simulink model "DegradationParameterIResistor"  (R2021a)
settings: Solver=VariableStepAuto  StartTime=0.0  StopTime=10.0  RelTol=1e-3
undefined symbols (not defined in the file or in its folder): Ires_resistance_adjustment
libraries: PB_Library_Master_Working x2
settings Model: Creator=sfaulk  LastModifiedBy=sfaulk

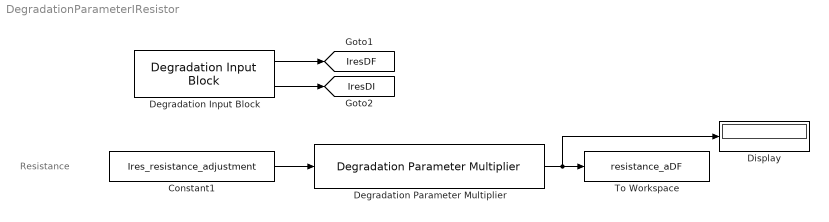
== system DegradationParameterIResistor ==
  note: Resistance
  Constant1 : Constant  Value=Ires_resistance_adjustment
  Degradation Input Block : PB_Library_Master_Working/Degradation Input Block  SystemSampleTime=-1  VariantActivationTime=update diagram  Latency=0  AutoFrameSizeCalculation=off
      link override Degradation Input Value: Value=Ires_degradation_input
  Degradation Parameter Multiplier : PB_Library_Master_Working/Degradation Parameter Multiplier  SystemSampleTime=-1  VariantActivationTime=update diagram  Latency=0  AutoFrameSizeCalculation=off
      link override From14: GotoTag=IresDF
      link override From15: GotoTag=IresDI
  Display : Display
  To Workspace : ToWorkspace  VariableName=resistance_aDF  SaveFormat=Timeseries  SampleTime=-1
      settings: Save2DSignal=2-D array (concatenate along first dimension)
  tag scope: IresDF=global, IresDI=global
  wires:
  Constant1/1 -> Degradation Parameter Multiplier/1
  Degradation Parameter Multiplier/1 -> Display/1, To Workspace/1
  Degradation Input Block/2 -> [IresDI]
  Degradation Input Block/1 -> [IresDF]
